simulink model "sim_all"  (R2020a)
settings: Solver=VariableStepAuto  StartTime=0.0  StopTime=2000  RelTol=1e-3
values from neighbouring files (symbols this model uses):
  a1 = rho * D^4 * alpha1    (= 0.000388302366464)    [data_current.m]
  a2 = -rho * D^3 * alpha2 * (1 - omega)    (= 0.0037030698432)    [data_current.m]
  alpha1 = 0.0113    [data_current.m]
  alpha2 = -0.0091    [data_current.m]
  cornerA = [43.781381 ... (first row only)    [missionC.m]
  cornerB = [43.780975 ... (first row only)    [missionC.m]
  cornerC = [43.780189 ... (first row only)    [missionC.m]
  cornerD = [43.780602 ... (first row only)    [missionC.m]
  ctrl_clockwise = false    [controller.m]
  ctrl_int_bound_or = 0.1    [controller.m]
  ctrl_int_bound_pos = 1    [controller.m]
  ctrl_k_or = 1    [controller.m]
  ctrl_k_pos = 1/3    (= 0.333333333333)    [controller.m]
  ctrl_Ki_vel = 100    [controller.m]
  ctrl_Kp_v_pos = 200    [controller.m]
  ctrl_Kp_vel = 200    [controller.m]
  ctrl_TAM = [  1     1           0           0               0       0;               0     0           1           1               0       0;               0     0           0           0               1       1;               0     0  -(ctrl_r+ctrl_dc)  ctrl_r+ctrl_dc    0       0;               0     0           0           0            -ctrl_r    ctrl_r;           -ctrl_r ctrl_r        0           0       ...(+19 chars)    [controller.m]
  ctrl_Ts = 0.1    [controller.m]
  ctrl_va_uncontrolled = 0.15    [controller.m]
  ctrl_vel_uncontrolled = 0.5    [controller.m]
  D = 0.076    [data_current.m]
  dead_zone_limit = 31.5    [data_current.m]
  depth = 5    [missionC.m]
  distanceFromWall = 8    [missionC.m]
  initInspectedSide = 2    [missionC.m]
  initPoint = [ 43.780796 ... (first row only)    [missionC.m]
  mod_A = pi*mod_R*mod_R    [model.m]
  mod_Cd_F = 0.45    [model.m]
  mod_Cd_M = 0.4    [model.m]
  mod_eta_init = [mod_xNorth; mod_yEast; -mod_zDown; 0; 0; 0]    [model.m]
  mod_g = 9.81    [model.m]
  mod_h0 = 0    [model.m]
  mod_Ixx = mod_Io(1,1)    [model.m]
  mod_Iyy = mod_Io(2,2)    [model.m]
  mod_Izz = mod_Io(3,3)    [model.m]
  mod_Kp_dot = 0    [model.m]
  mod_lat0 = 43.780189    [model.m]
  mod_lon0 = 11.282698    [model.m]
  mod_m = 100    [model.m]
  mod_Mq_dot = mod_Kp_dot    (= 0)    [model.m]
  mod_ni_init = [0; 0; 0; 0; 0; 0]    [model.m]
  mod_Nr_dot = mod_Kp_dot    (= 0)    [model.m]
  mod_p1 = [0; mod_R; 0]    [model.m]
  mod_p2 = [0; -mod_R; 0]    [model.m]
  mod_p3 = [0; 0; (mod_R + mod_z_cm)]    [model.m]
  mod_p4 = [0; 0; -(mod_R + mod_z_cm)]    [model.m]
  mod_p5 = [mod_R; 0; 0]    [model.m]
  mod_p6 = [-mod_R; 0; 0]    [model.m]
  mod_R = ((3*mod_Vol)/(4*pi))^(1/3)    [model.m]
  mod_Rm = (4*mod_R)/(3*pi)    [model.m]
  mod_t1 = [1; 0; 0]    [model.m]
  mod_t2 = [1; 0; 0]    [model.m]
  mod_t3 = [0; 1; 0]    [model.m]
  mod_t4 = [0; 1; 0]    [model.m]
  mod_t5 = [0; 0; 1]    [model.m]
  mod_t6 = [0; 0; 1]    [model.m]
  mod_W = mod_m*mod_g    (= 981)    [model.m]
  mod_Xu_dot = (2/3)*mod_rho_AUV*pi*(mod_R^3)    [model.m]
  mod_Yv_dot = mod_Xu_dot    [model.m]
  mod_z_cm = mod_r_cm(3)    [model.m]
  mod_Zw_dot = mod_Xu_dot    [model.m]
  n_max = 340    [data_current.m]
  nav_DT = 0.1    [navigation.m]
  nav_filter = -1    [data_analysis_simulation_total.m]    (also in navigation.m)
  nav_giro = 2    [navigation.m]
  nav_h0 = 0    [navigation.m]
  nav_lat0 = cornerC(1)    [navigation.m]
  nav_lon0 = cornerC(2)    [navigation.m]
  nav_plane_AB = coefficient_plane(nav_A,nav_B)    [navigation.m]
  nav_plane_BC = coefficient_plane(nav_B,nav_C)    [navigation.m]
  nav_plane_CD = coefficient_plane(nav_C,nav_D)    [navigation.m]
  nav_plane_DA = coefficient_plane(nav_D,nav_A)    [navigation.m]
  nav_resampling = 10000    [navigation.m]
  omega = 0.1    [data_current.m]
  relativeDirection = 30    [missionC.m]
  res_enable_n_eff = 1    [navigation.m]
  rho = 1030    [data_current.m]
  sens_distCM = 0.267    [sensors.m]
  sens_Sample_time_AHRS = 0.1    [sensors.m]
  sens_Sample_time_depth = 0.1    [sensors.m]
  sens_Sample_time_dvl = 0.2    [sensors.m]
  sens_Sample_time_GPS = 1    [sensors.m]
  sens_Sample_time_GYRO = 0.1    [sensors.m]
  sens_Sample_time_sonar = 0.5    [sensors.m]
  sens_threshold = 0.485    [sensors.m]
  sens_Variance_AHRS_pitch = (0.0087)^2    (= 7.569e-05)    [sensors.m]
  sens_Variance_AHRS_roll = (0.0087)^2    (= 7.569e-05)    [sensors.m]
  sens_Variance_AHRS_yaw = (0.0017)^2    (= 2.89e-06)    [sensors.m]
  sens_Variance_depth1 = (0.2)^2    (= 0.04)    [sensors.m]
  sens_Variance_depth2 = (0.4)^2    (= 0.16)    [sensors.m]
  sens_Variance_DVL = (speed*0.03)^2    [sensors.m]
  sens_Variance_GPS = 3    [sensors.m]
  sens_Variance_GYRO = 2.5133e-06    [sensors.m]
  sens_Variance_sonar = 0.05    [sensors.m]
  soglia_or = [0.1, 0.1, 0.1]    [mission.m]
  soglia_orp = 0.1    [mission.m]
  soglia_parete = 0.5    [mission.m]
  soglia_parete_frenata = 0.5    [mission.m]
  soglia_pos = [0.00001, 0.00001, 0.5]    [mission.m]
  soglia_SOS_collisione = 2    [mission.m]
  soglia_SOS_or = [0.25, 0.25, 0.25]    [mission.m]
  soglia_SOS_orp = 0.25    [mission.m]
  soglia_SOS_parete = 1    [mission.m]
  soglia_SOS_pos = [0.00005, 0.00005, 1]    [mission.m]
  soglia_SOS_pos_ris = 2    [mission.m]
  soglia_SOS_vel = 0.2    [mission.m]
  SOS = 0    [mission.m]
  speed = 0.4    [missionC.m]
  stato = 100    [mission.m]
  timer = 40*2    (= 80)    [mission.m]
  Ts_supervisor = 0.1    [mission.m]
undefined symbols (not defined in the file or in its folder): DiscIntNeverNeededParam, nav_A, nav_B, nav_C, nav_D
libraries: simulink x8, cstblocks x6, simulink_extras x1
(part 6 of 8)

== matlab function sim_all/Mission_supervisor_v3/Mission_Supervisor/Manovra/MATLAB Function ==
  data: delta_current_man output; delta_stato_man output; contatore output; contatore input; Pos_d output size=3; Dpp_d output; Dps_d output; Orp_d output; Pos_s input; Dpp_s input; Orp_s input; distanceFromWall parameter; relativeDirection parameter; depth parameter; error_flag input; soglia_orp parameter; soglia_SOS_parete parameter; soglia_SOS_pos parameter; SOS parameter; Dps_s input; alfa input; giro input; parete_attuale input
function [delta_current_man, delta_stato_man, contatore, Pos_d, Dpp_d, Dps_d, Orp_d] = Manovra(contatore, Pos_s, Dpp_s, Orp_s, distanceFromWall, relativeDirection, depth, error_flag, soglia_orp, soglia_SOS_parete, soglia_SOS_pos, SOS, Dps_s, alfa, giro, parete_attuale)

    disp("Manovra");
    
    %% Unità di misura 
     
    % Pos_d, Pos_s, soglia_SOS_pos                                                [deg,deg,m]
    % Orp_d, Orp_s, soglia_orp, alfa                                              [rad]
    % relativeDirection                                                           [deg]
    % Dpp_d, Dps_d, Dpp_s, Dps_s, distanceFromWall, depth, soglia_SOS_parete      [m]


    %% Inizializzazione variabili
    
    delta_stato_man = -2 * contatore;
    
    pronti = false;
    
    relativeDirection_rad = deg2rad(relativeDirection);
    
    % Si utilizza la variabile booleana giro, inizializzata nella matlab function "aggiornamento della parete"
    % per determinare il senso di pattugliamento
    if giro == 0 % orario
        inspectionDirection = "clockwise";
    else % antiorario
        inspectionDirection = "counterclockwise";
    end

    %% Preparazione dei riferimenti da fornire si blocchi successivi
          
    Pos_d = [nan; nan; depth];
                                                                            %*****TEST******%
                                                                            %Pos_d = [nan; nan; 0];
    % Distanza dalla parete da mantenere
    Dpp_d = distanceFromWall;
    Dps_d = distanceFromWall;
    
    % Orientazione relativa alla parete
    Orp_d = relativeDirection_rad;
    
    % In questo stato il riferimento di orientazione passato al controllo
    % si riferisce alla parete successiva. Questo rende necessario
    % l'introduzione della variabile "Orp_rif" utilizzata nelle condizioni
    % di switch poiché il valore di stima si riferisce ancora alla parete attuale.
    % I valori alfa corrispondono agli angoli interni ai corner del bacino.
    if (strcmp(inspectionDirection,'clockwise') == 1) % AB-BC-CD-DA
        
        if parete_attuale == 1 % pattugliamento AB, manovra in B
            Orp_rif = relativeDirection_rad + alfa(2); 
        elseif parete_attuale == 2 % pattugliamento BC, manovra in C
            Orp_rif = relativeDirection_rad + alfa(3);
        elseif parete_attuale == 3 % pattugliamento CD, manovra in D
            Orp_rif = relativeDirection_rad + alfa(4);
        else  % pattugliamento DA, manovra in A
            Orp_rif = relativeDirection_rad + alfa(1);
        end
        
    else % AB-DA-CD-BC
        
        if parete_attuale == 1 % pattugliamento AB, manovra in A
            Orp_rif = relativeDirection_rad - alfa(1);
        elseif parete_attuale == 2 % pattugliamento BC, manovra in B
            Orp_rif = relativeDirection_rad - alfa(2);
        elseif parete_attuale == 3 % pattugliamento CD, manovra in C
            Orp_rif = relativeDirection_rad - alfa(3);
        else % pattugliamento DA, manovra in D
            Orp_rif = relativeDirection_rad - alfa(4);
        end
    end
      
    % Transizione di stato effettiva
    delta_current_man = 203 - 202 + contatore;           
    
       
    %% Verifiche
    
    % Verifica di aver mantenuto la corretta profondità e distanza
    % dalle pareti considerate
    if (abs(Pos_s(3) - Pos_d(3)) > soglia_SOS_pos(3) || ...
       abs(Dpp_s - Dpp_d) > soglia_SOS_parete || ...
       abs(Dps_s - Dps_d) > soglia_SOS_parete)
    
        SOS = 1;
        disp("EMERGENZA:");
        
        if (abs(Pos_s(3) - Pos_d(3)) > soglia_SOS_pos(3))
            disp("Rilevato errore sulla profondita");
        end
        if (abs(Dpp_s - Dpp_d) > soglia_SOS_parete)
            disp("Rilevato errore sulla distanza da parete");
        end
        if (abs(Dps_s - Dps_d) > soglia_SOS_parete)
            disp("Rilevato errore sulla distanza da parete successiva");
        end
    end
    
                                                                            %*****TEST******%
                                                                            % if(contatore > 1)
                                                                            %     error_flag = 1;
                                                                            % end

     if error_flag == 1
        disp("EMERGENZA: errore segnalato dagli altri sottosistemi");
        SOS = 1;
     end
     
     
                                                                            %*****TEST******%
                                                                            %Serve per testare di rimanere 
                                                                            %in attesa in questo stato 
                                                                            %test = 0;
                                                                            %if(contatore > 2)%test
                                                                            %    test = 100;
                                                                            %else
                                                                            %    test = 0;
                                                                            %end
                                                                            
    % Si verifica di aver raggiunto l'orientazione desiderata 
    if (SOS == 0 && ...
        abs(Orp_s - Orp_rif) < soglia_orp)    
    
        pronti = true;
        
    end
    
    % La parete viene aggiornata soltanto
    % al termine della fase di manovra incrementando il contatore
    if pronti == true
         contatore = contatore + 1;
    end
    
     
    %% Decisione dello stato successivo
    
    if pronti == true
        if contatore < 4    % Non è ancora il pattugliamento dell'ultima parete 
            
            delta_stato_man = 201 - 203 - 2 * contatore +2;   % Si continua il pattugliamento delle pareti successive  
            
        else    % Completato il pattugliamento dell'ultima parete intera, si esce dal ciclo per
                % effettuare il pattugliamento parziale della parete
                % iniziale che era stata pattugliata solo per metà
                
            delta_stato_man = 204-203 - 2 * contatore +2;         
        end
    end
    
    if SOS == 1
            
            delta_stato_man = 301-203 + - 2 * contatore; %Transizione nello stato di emergenza
    end
        % Si rimane nello stato corrente

end

== matlab function sim_all/Mission_supervisor_v3/Mission_Supervisor/Completamento/MATLAB Function ==
  data: delta_current_comp output; parete input; delta_stato_comp output; Pos_d output size=3; Vel_d output; Dpp_d output; Orp_d output; Pos_s input; Vel_s input; Dpp_s input; Dps_s input; Orp_s input; depth parameter; speed parameter; distanceFromWall parameter; relativeDirection parameter; dps_fin input; error_flag input; soglia_SOS_vel parameter; soglia_parete_frenata parameter; soglia_SOS_orp parameter; soglia_SOS_pos parameter; soglia_SOS_parete parameter; SOS parameter; giro input
function [delta_current_comp, delta_stato_comp, Pos_d, Vel_d, Dpp_d, Orp_d] = Completamento(parete, Pos_s, Vel_s, Dpp_s, Dps_s, Orp_s, depth, speed, distanceFromWall, relativeDirection, dps_fin, error_flag, soglia_SOS_vel, soglia_parete_frenata, soglia_SOS_orp, soglia_SOS_pos, soglia_SOS_parete, SOS, giro)

    disp("Completamento del pattugliamento parziale della parete " + parete);
    
    %% Unità di misura 
    
    % Pos_d, Pos_s, soglia_SOS_pos                                                                              [deg, deg, m]
    % Orp_d, Orp_s, soglia_SOS_orp                                                                              [rad]
    % relativeDirection                                                                                         [deg]
    % Dpp_d, Dps_d, Dpp_s, Dps_s, dps_fin, distanceFromWall, depth, soglia_SOS_parete, soglia_parete_frenata    [m]
    % Vel_d, Vel_s, speed, soglia_SOS_vel                                                                       [m/s]

    %% Inizializzazione variabili
    
    % Utilizzata per permanere in questo stato e inizializzata a zero
    % perché fuori dal ciclo
    delta_stato_comp = 0; 
    
    pronti = false;
    
    
    %% Preparazione dei riferimenti da fornire ai blocchi successivi
    
    % Profondità da mantenere
    Pos_d = [nan; nan; depth];
                                                                            %*****TEST******%
                                                                            %Pos_d = [nan; nan; 0];
    
    % Velocità da raggiungere
    Vel_d = speed;              
                                                                            %*****TEST******%
                                                                            %Vel_d_vett = [0; 0; 0];

    % Distanza dalla parete da mantenere
    Dpp_d = distanceFromWall;
    
    % Orientazione da mantenere
    Orp_d = deg2rad(relativeDirection);
        
    % Transizione di stato effettiva
    delta_current_comp = 204 - 203;  
  
    %% Verifiche
    
    % Verifica sulla corretta profondità, orientazione, distanza dalla parete pattugliata 
    % e velocità
    if (abs(Pos_s(3) - Pos_d(3)) > soglia_SOS_pos(3) || ...
        abs(Orp_s - Orp_d) > soglia_SOS_orp || ...
        abs(Dpp_s - Dpp_d) > soglia_SOS_parete || ...
        norm(Vel_s) - Vel_d > soglia_SOS_vel)
    
        SOS = 1;
        disp("EMERGENZA:");
        
        if (abs(Orp_s - Orp_d) > soglia_SOS_orp)
            disp("Rilevato errore sull'orientazione relativa");
        end
        
        if (abs(Dpp_s - Dpp_d) > soglia_SOS_parete)
            disp("Rilevato errore sulla distanza da parete");
        end
        
        if (abs(Pos_s(3) - Pos_d(3)) > soglia_SOS_pos(3))
            disp("Rilevato errore sulla profondita Z");
        end
        
        if (norm(Vel_s) - Vel_d > soglia_SOS_vel)
            disp("Rilevato errore nella velocita");
        end

    end
    
                                                                            %*****TEST******%
                                                                            % if(contatore > 1)
                                                                            %     error_flag = 1;
                                                                            % end

     if error_flag == 1
        disp("EMERGENZA: errore segnalato dagli altri sottosistemi");
        SOS = 1;
     end
     
                                                                            %*****TEST******%
                                                                            %dps_fin = 4;

    % Si verifica di pattugliare alla velocità desiderata fino al punto di
    % frenata
    if (SOS == 0 && ...
        abs(Dps_s - (dps_fin + 3*speed)) < soglia_parete_frenata) % Analogo a quanto detto in "Pattugliamento"
    
        pronti = true;
        
    end
    
    %% Decisione dello stato successivo
    
    if pronti == true
        
        delta_stato_comp = 205 - 204; % Transizione eseguita correttamente
    end
    if SOS == 1
            
            delta_stato_comp = 301 - 204; % Transizione nello stato di emergenza
    end
  % Si rimane nello stato corrente.

end

== matlab function sim_all/Mission_supervisor_v3/Mission_Supervisor/Frenata in completamento/MATLAB Function ==
  data: delta_current_fren_comp output; delta_stato_fren_comp output; SOS_205 output; Pos_d output size=3; Dpp_d output; Dps_d output; Orp_d output; Pos_s input; Orp_s input; Dpp_s input; Dps_s input; depth parameter; distanceFromWall parameter; relativeDirection parameter; dps_fin input; error_flag input; soglia_SOS_pos parameter; soglia_SOS_parete parameter; soglia_SOS_orp parameter; soglia_parete parameter; SOS parameter
function [delta_current_fren_comp, delta_stato_fren_comp, SOS_205, Pos_d, Dpp_d, Dps_d, Orp_d] = Frenata_completamento(Pos_s, Orp_s, Dpp_s, Dps_s, depth, distanceFromWall, relativeDirection, dps_fin, error_flag, soglia_SOS_pos, soglia_SOS_parete, soglia_SOS_orp, soglia_parete, SOS)

    disp("Frenata (durante il completamento del pattugliamento parziale)");
    
    %% Unità di misura 
    
    % Pos_d, Pos_s, soglia_SOS_pos                                                                      [deg, deg, m]
    % Orp_d, Orp_s, soglia_SOS_orp                                                                      [rad]
    % relativeDirection                                                                                 [deg]
    % Dpp_d, Dps_d, Dpp_s, Dps_s, dps_fin, distanceFromWall, depth, soglia_SOS_parete, soglia_parete    [m]
    
    %% Inizializzazione variabili
    
    delta_stato_fren_comp = 0;
    
    pronti = false;
    

    %% Preparazione dei riferimenti da fornire si blocchi successivi
    
    % Profondità da mantenere
    Pos_d = [nan; nan; depth];
                                                                            %*****TEST******%
                                                                            %Pos_d = [nan;nan;0];
    % Distanza dalla parete da mantenere
    Dpp_d = distanceFromWall;
    Dps_d = dps_fin;
    
    % Orientazione da mantenere
    Orp_d = deg2rad(relativeDirection);
    
    % Transizione di stato effettiva
    delta_current_fren_comp = 205 - 204;  
    
       
    %% Verifiche

    % Si verifica la corretta orientazione, profondità e distanza dalla parete di pattugliamento 
    if (abs(Pos_s(3) - Pos_d(3)) > soglia_SOS_pos(3) || ...
        abs(Orp_s - Orp_d) > soglia_SOS_orp || ...
        abs(Dpp_s - Dpp_d) > soglia_SOS_parete)
    
        SOS = 1;
        pronti = true;
        disp("EMERGENZA:");
        
        if (abs(Pos_s(3) - Pos_d(3)) > soglia_SOS_pos(3))
            disp("Rilevato errore sulla profondita Z");
        end
        
        if (abs(Orp_s - Orp_d) > soglia_SOS_orp)
            disp("Rilevato errore sull'orientazione relativa");
        end
        
        if (abs(Dpp_s - Dpp_d) > soglia_SOS_parete)
            disp("Rilevato errore sulla distanza da parete");
        end
    end
    
    if error_flag == 1
        disp("EMERGENZA: errore segnalato dagli altri sottosistemi");
        SOS = 1;
    end
 
    SOS_205 = SOS;                                                                     %*****TEST******%
                                                                            %dps_fin = 8;

    % Si verifica di aver raggiunto la posizione desiderata di fine pattugliamento
    if (SOS==0 && ...
        abs(Dps_s - dps_fin) < soglia_parete) 
        pronti = true;
        
    end
    
    %% Decisione dello stato successivo
    
    if (pronti == true || SOS == 1)
        
        delta_stato_fren_comp = 301 - 205; % Transizione di stato
    end
    % Si rimane nello stato corrente
    

end

== matlab function sim_all/Mission_supervisor_v3/Mission_Supervisor/Orientazione in superficie/MATLAB Function ==
  data: delta_current_or_sup output; delta_stato_or_sup output; Or_in input; error_flag input; punto_iniz_patt input; SOS parameter; Pos_d output size=3; Or_d output size=3; soglia_SOS_pos parameter; soglia_or parameter; Pos_s input; Or_s input; soglia_SOS_or parameter
function [delta_current_or_sup, delta_stato_or_sup, Pos_d, Or_d] = Orientazioneinsuperficie(Or_in, error_flag, punto_iniz_patt, SOS, soglia_SOS_pos, soglia_or, Pos_s, Or_s, soglia_SOS_or)

    disp("Orientazione in superficie");
    
    %% Unità di misura 
    
    % Pos_d, Pos_s, soglia_SOS_pos, punto_iniz_patt                             [deg,deg,m]
    % Or_d, Or_in, Or_s, soglia_SOS_or, soglia_or                               [deg,deg,deg]

    %% Inizializzazione variabili
    
    delta_stato_or_sup = 0;
    
    pronti = false; 

    %% Preparazione dei riferimenti da fornire ai blocchi successivi
  
    % Posizione da mantenere
    Pos_d = punto_iniz_patt; 
                                                                            %*****TEST******%
                                                                            %Pos_d = [43; 11; 0];  
    % Orientazione desiderata e necessaria per raggiungere
    % il punto di rientro
    Or_d = Or_in;
                                                                            %*****TEST******%
                                                                            %Or_d = [1; 1; 1];
  
    % Transizione di stato effettiva
    delta_current_or_sup = 302 - 301;
   
    
    %% Verifiche 
    
    % Verifica della posizione e dell'orientazione
   if (abs(Pos_s(1) - Pos_d(1)) > soglia_SOS_pos(1) || ...
       abs(Pos_s(2) - Pos_d(2)) > soglia_SOS_pos(2) || ...
       abs(Pos_s(3) - Pos_d(3)) > soglia_SOS_pos(3) || ...
       abs(Or_s(1) - Or_d(1)) > soglia_SOS_or(1) || ...
       abs(Or_s(2) - Or_d(2)) > soglia_SOS_or(2))
    
        SOS = 1;
        disp("EMERGENZA:");
        
        
        if (abs(Pos_s(1) - Pos_d(1)) > soglia_SOS_pos(1))
            disp("Rilevato errore sulla posizione X");
        end
        if (abs(Pos_s(2) - Pos_d(2)) > soglia_SOS_pos(2))
            disp("Rilevato errore sulla posizione Y");
        end
        if (abs(Pos_s(3) - Pos_d(3)) > soglia_SOS_pos(3))
            disp("Rilevato errore sulla profondita Z");
        end
        if (abs(Or_s(1) - Or_d(1)) > soglia_SOS_or(1))
            disp("Rilevato errore sulla rotazione di roll");
        end
        if (abs(Or_s(2) - Or_d(2)) > soglia_SOS_or(2))
            disp("Rilevato errore sulla rotazione di pitch");
        end

    end
    
    if error_flag == 1
        disp("EMERGENZA: errore segnalato dagli altri sottosistemi");
        SOS = 1;
    end
    
    % Si verifica di aver raggiunto l'orientazione desiderata
    if  (SOS == 0 && ...
         abs(Or_s(3) - Or_d(3)) < soglia_or(3))
    
        pronti = true;
        
    end
    
%% Decisione dello stato successivo
    
    if pronti == true
       
        delta_stato_or_sup = 303 - 302; % Transizione eseguita correttamente
    end
    
    if SOS == 1
            
            delta_stato_or_sup = 304 - 302; % Transizione nello stato di emergenza
    end

    % Si rimane nello stato corrente
end

== matlab function sim_all/Mission_supervisor_v3/Mission_Supervisor/Pattugliamento/MATLAB Function ==
  data: parete input; contatore input; delta_current_patt output; Pos_s input; Dpp_s input; Dps_s input; delta_stato_patt output; Pos_d output size=3; Vel_d output; Dpp_d output; Orp_d output; Orp_s input; Vel_s input; depth parameter; speed parameter; distanceFromWall parameter; relativeDirection parameter; soglia_parete_frenata parameter; soglia_SOS_orp parameter; soglia_SOS_parete parameter; soglia_SOS_pos parameter; error_flag input; SOS parameter; soglia_SOS_vel parameter; giro input
function [delta_current_patt, delta_stato_patt, Pos_d, Vel_d, Dpp_d, Orp_d] = Pattugliamento(parete, contatore, Pos_s, Dpp_s, Dps_s, Orp_s, Vel_s, depth, speed, distanceFromWall, relativeDirection, soglia_parete_frenata, soglia_SOS_orp, soglia_SOS_parete, soglia_SOS_pos, error_flag, SOS, soglia_SOS_vel, giro)
    
    % In base al valore del contatore un display mostra il tipo di pattugliamento (parziale o completo)
    if contatore == 0
        disp("Pattugliamento parziale parete " + parete);
    else
        disp("Pattugliamento parete " + parete);
    end 
    
    %% Unità di misura 
    
    % Pos_d, Pos_s, soglia_SOS_pos                                                        [deg, deg, m]
    % Orp_d, Orp_s, soglia_SOS_orp                                                        [rad]
    % relativeDirection                                                                   [deg]
    % Dpp_d,Dpp_s, depth, distanceFromWall, soglia_parete_frenata, soglia_SOS_parete      [m]
    % Vel_d, Vel_s, speed, soglia_SOS_vel                                                 [m/s]

    
    %% Inizializzazione variabili
    
    % Si attribuisce alla variabile delta_stato_patt il valore contatore per  
    % tenere traccia delle transizioni effettuate durante il ciclo di
    % pattugliamento. Questo deve essere fatto perché i valori delta_stato
    % rimangono attivi una volta inizializzati nel ciclo.
    delta_stato_patt = contatore;
    
    pronti = false;
    
    %% Preparazione dei riferimenti da fornire ai blocchi successivi
    
    % Profondità da mantenere
    Pos_d = [nan; nan; depth];
                                                                            %*****TEST******%
                                                                            %Pos_d = [nan;nan;0];
    
    % Velocità da raggiungere
    Vel_d = speed;             

    % Distanza dalla parete da mantenere
    Dpp_d = distanceFromWall;
    
    % Orientazione da mantenere
    Orp_d = deg2rad(relativeDirection);
    
    
    % Transizione di stato effettiva a seconda che si arrivi da
    % "Orientazione in profondità" o da "Manovra"
    delta_current_patt = 201-104;   
   
    if contatore>0
        delta_current_patt = 201 - 104 - (2*contatore); 
    end
       
    %% Verifiche
    
    %Verifica sull'orientazione, sulla velocità, sulla profondità e sulla
    %distanza dalla parete pattugliata
    if (abs(Pos_s(3) - Pos_d(3)) > soglia_SOS_pos(3) || ...
        abs(Orp_s - Orp_d) > soglia_SOS_orp || ...
        norm(Vel_s) - Vel_d > soglia_SOS_vel || ...
        abs(Dpp_s - Dpp_d) > soglia_SOS_parete)
 
        SOS = 1;
        disp("EMERGENZA:");
        
        if (abs(Orp_s-Orp_d) > soglia_SOS_orp)
            disp("Rilevato errore sull'orientazione relativa");
        end
        if (abs(Dpp_s - Dpp_d) > soglia_SOS_parete)
            disp("Rilevato errore sulla distanza da parete");
        end
        if (abs(Pos_s(3) - Pos_d(3)) > soglia_SOS_pos(3))
            disp("Rilevato errore sulla profondita");
        end
        if (norm(Vel_s) - Vel_d > soglia_SOS_vel)
            disp("Rilevato errore sulla velocita");
        end

    end
%                                                                             %*****TEST******%
%                                                                             if(contatore>1)
%                                                                                 error_flag=1;
%                                                                             end

     if error_flag == 1
        disp("EMERGENZA: errore segnalato dagli altri moduli");
        SOS = 1;
     end
                                                                            %*****TEST******%
                                                                            %Serve per testare di rimanere 
                                                                            %in attesa in questo stato 
                                                                            %test=0;
%                                                                             if(contatore>1)%test
%                                                                                test=100;
%                                                                             else
%                                                                                test=0;
%                                                                             end
    
    % Si verifica di pattugliare fino al punto di frenata calcolata
    % considerando un tempo di frenata di tre secondi
    if (SOS == 0 && ...
        abs(Dps_s - (distanceFromWall + 3*speed)) < soglia_parete_frenata) 

        
        pronti = true;
        
    end
    
    %% Decisione dello stato successivo
    
    if pronti == true

        delta_stato_patt = 202 - 201 + contatore; %Transizione eseguita correttamente
    end
    if SOS == 1
            
            delta_stato_patt = 301 - 201 + contatore; %Transizione nello stato di emergenza
    end
% Si rimane nello stato corrente

end

== matlab function sim_all/Mission_supervisor_v3/Mission_Supervisor/Fine missione/MATLAB Function ==
  data: delta_current_end output; stato input
function delta_current_end  = Fine_missione(stato)

    disp("Fine missione");
    
    
    
    %% Transizione di stato effettiva 
    delta_current_end = 304 - stato;  
    
    % La missione è conclusa e la simulazione termina.

end

== matlab function sim_all/Mission_supervisor_v3/Mission_Supervisor/Posizionamento/MATLAB Function ==
  data: delta_current_posiz output; delta_stato_posiz output; Pos_d output size=3; Or_d output size=3; Pos_s input; Or_s input; punto_iniziale input; Or_in input; error_flag input; soglia_pos parameter; soglia_SOS_or parameter; SOS parameter; soglia_SOS_pos parameter
function [delta_current_posiz, delta_stato_posiz, Pos_d, Or_d] = Posizionamento(Pos_s, Or_s, punto_iniziale, Or_in, error_flag, soglia_pos, soglia_SOS_or, SOS, soglia_SOS_pos)

    disp("Posizionamento");
    
    %% Unità di misura 
    
    % Pos_d, Pos_s, punto_iniziale, soglia_pos, soglia_SOS_pos             [deg, deg, m]
    % Or_d, Or_s, Or_in, soglia_SOS_or                                     [rad, rad, rad]

    %% Inizializzazione variabili
    
    % Mantenimento dello stato_interno al valore
    % desiderato durante la permanenza del sistema nello stato corrente.
    delta_stato_posiz = 0;
    
    pronti = false;
   
    %% Preparazione dei riferimenti da fornire ai blocchi successivi
    
    % Posizione da raggiungere
    Pos_d = punto_iniziale;                                                %*****TEST******%
                                                                            %Pos_d = [43; 11; 0];
     
   
    % Orientazione da mantenere
    Or_d = Or_in;
    
    % Transizione di stato effettiva
    delta_current_posiz = 102 - 101;  
       
    
    %% Verifiche
    
     % Verifica della corretta orientazione e profondità
     
    if (abs(Or_s(1) - Or_d(1)) > soglia_SOS_or(1) || ...
        abs(Or_s(2) - Or_d(2)) > soglia_SOS_or(2) || ...
        abs(Or_s(3) - Or_d(3)) > soglia_SOS_or(3) || ...
        abs(Pos_s(3) - Pos_d(3)) > soglia_SOS_pos(3))
    
        SOS = 1;
        disp("EMERGENZA:");       
        
        if (abs(Or_s(1) - Or_d(1)) > soglia_SOS_or(1))
            disp("Rilevato errore sulla rotazione di roll");
        end
        
        if (abs(Or_s(2) - Or_d(2)) > soglia_SOS_or(2))
            disp("Rilevato errore sulla rotazione di pitch");
        end
        
        if (abs(Or_s(3) - Or_d(3)) > soglia_SOS_or(3))
            disp("Rilevato errore sulla rotazione di yaw");
        end
       
        if (abs(Pos_s(3) - Pos_d(3)) > soglia_SOS_pos(3))
            disp("Rilevato errore sulla posizione lungo z");
        end
        
    end
    
    if error_flag == 1
        disp("EMERGENZA: errore segnalato dagli altri sottosistemi");
        SOS = 1;
    end
    
    % Si verifica di aver raggiunto la posizione desiderata
    if (SOS == 0 && ...
        abs(Pos_s(1) - Pos_d(1)) < soglia_pos(1) && ...
        abs(Pos_s(2) - Pos_d(2)) < soglia_pos(2))
    
        pronti = true;
        
    end

    %% Decisione dello stato successivo
     
    if pronti == true
        
        delta_stato_posiz = 103 - 102; % Transizione eseguita correttamente
    end
    if SOS == 1
            
            delta_stato_posiz = 304 - 102; % Transizione nello stato di emergenza
    end
    % Si rimane nello stato corrente

end

== matlab function sim_all/Mission_supervisor_v3/Mission_Supervisor/Rientro/MATLAB Function ==
  data: delta_current_rient output; delta_stato_rient output; Pos_d output size=3; Pos_s input; initPoint parameter; Or_in input; Or_d output size=3; soglia_pos parameter; SOS parameter; error_flag input; Dps_s input; Dpp_s input; soglia_SOS_collisione parameter; soglia_SOS_or parameter; soglia_SOS_pos parameter; Or_s input
function [delta_current_rient, delta_stato_rient, Pos_d, Or_d] = Rientro(Pos_s, initPoint, Or_in, soglia_pos, SOS, error_flag, Dps_s, Dpp_s, soglia_SOS_collisione, soglia_SOS_or, soglia_SOS_pos, Or_s)

    disp("Rientro");
    
    %% Unità di misura 
    
    % Pos_d, Pos_s, soglia_pos, initPoint, soglia_SOS_pos                    [deg,deg,m]
    % Or_d, Or_in, Or_s, soglia_SOS_or                                       [deg,deg,deg]
    % Dps_s, Dpp_s, soglia_SOS_collisione_s                                  [m]

    %% Inizializzazione variabili
    
    delta_stato_rient = 0;
    
    pronti = false;
    
    %% Preparazione dei riferimenti da fornire ai blocchi successivi
      
    % Posizione da raggiungere
    Pos_d = initPoint;
    
    % Orientazione da mantenere
    Or_d = Or_in;
    
    % Transizione di stato effettiva
    delta_current_rient = 303 - 302; 
       
    %% Verifiche
    
    % Verifica sulla profondità, sull'orientazione e sull'assenza di collisioni
    if (Dpp_s  < soglia_SOS_collisione || ... 
        Dps_s < soglia_SOS_collisione || ...
        abs(Or_s(1) - Or_d(1)) > soglia_SOS_or(1) || ...
        abs(Or_s(2) - Or_d(2)) > soglia_SOS_or(2) || ...
        abs(Or_s(3) - Or_d(3)) > soglia_SOS_or(3) || ...
        abs(Pos_s(3) - Pos_d(3)) > soglia_SOS_pos(3))
            
    
        SOS = 1;
        disp("EMERGENZA:");  
 

        if (Dpp_s < soglia_SOS_collisione || ... 
            Dps_s < soglia_SOS_collisione)
            disp("Pericolo collisione");
        end
        
        if (abs(Or_s(1) - Or_d(1)) > soglia_SOS_or(1))
            disp("Rilevato errore sulla rotazione di roll");
        end
        
        if (abs(Or_s(2) - Or_d(2)) > soglia_SOS_or(2))
            disp("Rilevato errore sulla rotazione di pitch");
        end
        
        if (abs(Or_s(3) - Or_d(3)) > soglia_SOS_or(3))
            disp("Rilevato errore sulla rotazione di yaw");
        end
     
        if (abs(Pos_s(3) - Pos_d(3)) > soglia_SOS_pos(3))
            disp("Rilevato errore sulla posizione lungo z");
        end
    
    end
    
    if error_flag == 1
        
        disp("EMERGENZA: errore segnalato dagli altri sottosistemi");
        SOS = 1;
        
    end
   
    % Si verifica di aver raggiunto la posizione desiderata
    if (SOS == 0 && ...
        abs(Pos_s(1) - Pos_d(1)) < soglia_pos(1) && ...
        abs(Pos_s(2) - Pos_d(2)) < soglia_pos(2))
    
        pronti = true;
        
    end
    

    
   %% Decisione dello stato successivo
    
   % Si effettua la transizione nello stato successivo indipendentemente
   % dal verificarsi di una emergenza
    if (pronti == true || SOS == 1)

        delta_stato_rient = 304 - 303;
    end
    % Si rimane nello stato corrente

end

== matlab function sim_all/PF/Calcolo distaza pareti/Calcolo distanza dalle pareti ==
  data: pos_es input; dpp output; dps output; parete_attuale input; nav_plane_AB parameter; nav_plane_BC parameter; nav_plane_CD parameter; nav_plane_DA parameter; nav_giro parameter
% Applicando la formula della distanza di un punto da un piano ottengo la
% distanza della posizione dell'AUV dalla parete d'interesse. 

function [dpp,dps] = dpp_dps_calculator(pos_es, parete_attuale, nav_plane_AB, nav_plane_BC, nav_plane_CD, nav_plane_DA, nav_giro)
    
%selezione della parete di pattugliamento e successiva
    switch parete_attuale
        
        case 1
           coef = nav_plane_AB;            %parete attuale AB
           if nav_giro == 1
               coef_succ = nav_plane_BC;   %parete succ BC
           else
               coef_succ = nav_plane_DA;   %parete succ DA
           end
           
        case 2
           coef = nav_plane_BC;            %parete attuale BC
           if nav_giro == 1
               coef_succ = nav_plane_CD;   %parete succ CD
           else
               coef_succ = nav_plane_AB;   %parete succ AB
           end
           
        case 3
           coef = nav_plane_CD;            %parete attuale CD
           if nav_giro == 1
               coef_succ = nav_plane_DA;   %parete succ DA
           else
               coef_succ = nav_plane_BC;   %parete succ BC
           end
        case 4
           coef = nav_plane_DA;            %parete attuale DA
           if nav_giro == 1
               coef_succ = nav_plane_AB;   %parete succ AB
           else
               coef_succ = nav_plane_CD;   %parete succ CD
           end
        otherwise
            coef = [0 0 0 0];
            coef_succ = [0 0 0 0];
    end

    dpp = abs(coef(1)*pos_es(1)+coef(2)*pos_es(2)-coef(3)*pos_es(3)+coef(4))/norm([coef(1) coef(2) coef(3)]);
    dps = abs(coef_succ(1)*pos_es(1)+coef_succ(2)*pos_es(2)-coef_succ(3)*pos_es(3)+coef_succ(4))/norm([coef_succ(1) coef_succ(2) coef_succ(3)]);
   
end

== matlab function sim_all/PF/Calcolo distaza pareti/Calcolo orientazione dalla parete ==
  data: pos_es input; orient_parete output; parete_attuale input; orient input; nav_plane_AB parameter; nav_plane_BC parameter; nav_plane_CD parameter; nav_plane_DA parameter
function orient_parete  = orient_parete_calculator(pos_es, parete_attuale, orient, nav_plane_AB, nav_plane_BC, nav_plane_CD, nav_plane_DA)
    
    %consideriamo angoli di pitch e roll nulli, cioè calcoliamo
    %l'orientazione rispetto alla parete solo considerando rotazioni di yaw
    %(piano xy)

    Yaw   = orient(3);
    R_z = [cos(Yaw)     sin(Yaw)       0     ;
           -sin(Yaw)    cos(Yaw)       0     ;
              0            0           1    ];
    v_pos= R_z'*[1 0 0]';  %versore della retta lungo l'asse x (in body) in NED,
                       %cioè la direzione di riferimento di prua del veicolo     
    
    %selezione della parete di pattugliamento
switch parete_attuale                      
    case 1
        %% Piano di pattugliamento AB
        versore_plane_NED = [nav_plane_AB(1) nav_plane_AB(2) 0]';    %versore normale al piano
        versore_plane_NED = versore_plane_NED/norm(versore_plane_NED);

        %calcolo distanza e intersezione lungo la normale al piano
        t_ = -(pos_es(1)+nav_plane_AB(2)*pos_es(2)+nav_plane_AB(4))/(nav_plane_AB(2)*versore_plane_NED(2)+versore_plane_NED(1));
        inter_perp=zeros(3,1);
        inter_perp(1) = pos_es(1) + versore_plane_NED(1)*t_;
        inter_perp(2) = pos_es(2) + versore_plane_NED(2)*t_;
        inter_perp(3) = pos_es(3) + versore_plane_NED(3)*t_;
        
        %calcolo distanza e intersezione lungo la direzione di prua
        t_ = -(pos_es(1)+nav_plane_AB(2)*pos_es(2)+nav_plane_AB(4))/(nav_plane_AB(2)*v_pos(2)+v_pos(1));
        inter_prua=zeros(3,1);
        inter_prua(1) = pos_es(1) + v_pos(1)*t_;
        inter_prua(2) = pos_es(2) + v_pos(2)*t_;
        inter_prua(3) = pos_es(3) + v_pos(3)*t_;
        
        coef = nav_plane_AB;
        coef(4)=[];
        orient_parete = rad2deg(asin(abs(coef*v_pos)/(norm(coef)*norm(v_pos))));
        %se orient_parete è positiva, allora ci troviamo tra - 90 e + 90 rispetto alla normale della parete 
        if t_ > 0              
            if inter_prua(1) > inter_perp(1) && inter_prua(2) < inter_perp(2)
                orient_parete = orient_parete - 90;
            else
                orient_parete = -(orient_parete - 90);
            end
        else
            if inter_prua(1) > inter_perp(1) && inter_prua(2) < inter_perp(2)
                orient_parete = (orient_parete + 90);
            else
                orient_parete = -(orient_parete + 90);
            end
        end    
    case 2
        %% Piano di pattugliamento BC
      	versore_plane_NED = [nav_plane_BC(1) nav_plane_BC(2) 0]';    %versore normale al piano
        versore_plane_NED = versore_plane_NED/norm(versore_plane_NED);

        %calcolo distanza e intersezione lungo la normale al piano
        t_ = -(pos_es(1)+nav_plane_BC(2)*pos_es(2)+nav_plane_BC(4))/(nav_plane_BC(2)*versore_plane_NED(2)+versore_plane_NED(1));
        inter_perp=zeros(3,1);
        inter_perp(1) = pos_es(1) + versore_plane_NED(1)*t_;
        inter_perp(2) = pos_es(2) + versore_plane_NED(2)*t_;
        inter_perp(3) = pos_es(3) + versore_plane_NED(3)*t_;

        %calcolo distanza e intersezione lungo la direzione di prua
        t_ = -(pos_es(1)+nav_plane_BC(2)*pos_es(2)+nav_plane_BC(4))/(nav_plane_BC(2)*v_pos(2)+v_pos(1));
        inter_prua=zeros(3,1);
        inter_prua(1) = pos_es(1) + v_pos(1)*t_;
        inter_prua(2) = pos_es(2) + v_pos(2)*t_;
        inter_prua(3) = pos_es(3) + v_pos(3)*t_;
        
        coef = nav_plane_BC;
        coef(4)=[];
        v_pos=-v_pos;
        orient_parete = rad2deg(asin(abs(coef*v_pos)/(norm(coef)*norm(v_pos))));
        %se orient_parete è positiva, allora ci troviamo tra - 90 e + 90 rispetto alla normale della parete 
        if t_ > 0              
            if inter_prua(1) > inter_perp(1) && inter_prua(2) > inter_perp(2)
                orient_parete = orient_parete - 90;
            else
                orient_parete = -(orient_parete - 90);
            end
        else
            if inter_prua(1) > inter_perp(1) && inter_prua(2) > inter_perp(2)
                orient_parete = orient_parete + 90;
            else
                orient_parete = -(orient_parete + 90);
            end
        end
        
    case 3
        %% Piano di pattugliamento CD
      	versore_plane_NED = [nav_plane_CD(1) nav_plane_CD(2) 0]';    %versore normale al piano
        versore_plane_NED = versore_plane_NED/norm(versore_plane_NED);

        %calcolo distanza e intersezione lungo la normale al piano
        t_ = -(pos_es(1)+nav_plane_CD(2)*pos_es(2)+nav_plane_CD(4))/(nav_plane_CD(2)*versore_plane_NED(2)+versore_plane_NED(1));
        inter_perp=zeros(3,1);
        inter_perp(1) = pos_es(1) + versore_plane_NED(1)*t_;
        inter_perp(2) = pos_es(2) + versore_plane_NED(2)*t_;
        inter_perp(3) = pos_es(3) + versore_plane_NED(3)*t_;

        %calcolo distanza e intersezione lungo la direzione di prua
        t_ = -(pos_es(1)+nav_plane_CD(2)*pos_es(2)+nav_plane_CD(4))/(nav_plane_CD(2)*v_pos(2)+v_pos(1));
        inter_prua=zeros(3,1);
        inter_prua(1) = pos_es(1) + v_pos(1)*t_;
        inter_prua(2) = pos_es(2) + v_pos(2)*t_;
        inter_prua(3) = pos_es(3) + v_pos(3)*t_;
        
        coef = nav_plane_CD;
        coef(4)=[];
        v_pos=-v_pos;
        orient_parete = rad2deg(asin(abs(coef*v_pos)/(norm(coef)*norm(v_pos))));
        %se orient_parete è positiva, allora ci troviamo tra - 90 e + 90 rispetto alla normale della parete 
        if t_ > 0              
            if inter_prua(1) > inter_perp(1) && inter_prua(2) < inter_perp(2)
                orient_parete = -orient_parete + 90;
            else
                orient_parete = orient_parete - 90;
            end
        else
             if inter_prua(1) > inter_perp(1) && inter_prua(2) < inter_perp(2)
                orient_parete = -orient_parete - 90;
            else
                orient_parete = orient_parete + 90;
            end
        end
        
    case 4
        %% Piano di pattugliamento DA
      	versore_plane_NED = [nav_plane_DA(1) nav_plane_DA(2) 0]';    %versore normale al piano
        versore_plane_NED = versore_plane_NED/norm(versore_plane_NED);

        %calcolo distanza e intersezione lungo la normale al piano
        t_ = -(pos_es(1)+nav_plane_DA(2)*pos_es(2)+nav_plane_DA(4))/(nav_plane_DA(2)*versore_plane_NED(2)+versore_plane_NED(1));
        inter_perp=zeros(3,1);
        inter_perp(1) = pos_es(1) + versore_plane_NED(1)*t_;
        inter_perp(2) = pos_es(2) + versore_plane_NED(2)*t_;
        inter_perp(3) = pos_es(3) + versore_plane_NED(3)*t_;

        %calcolo distanza e intersezione lungo la direzione di prua
        t_ = -(pos_es(1)+nav_plane_DA(2)*pos_es(2)+nav_plane_DA(4))/(nav_plane_DA(2)*v_pos(2)+v_pos(1));
        inter_prua=zeros(3,1);
        inter_prua(1) = pos_es(1) + v_pos(1)*t_;
        inter_prua(2) = pos_es(2) + v_pos(2)*t_;
        inter_prua(3) = pos_es(3) + v_pos(3)*t_;
        
        coef = nav_plane_DA;
        coef(4)=[];
        orient_parete = rad2deg(asin(abs(coef*v_pos)/(norm(coef)*norm(v_pos))));
        %se orient_parete è positiva, allora ci troviamo tra - 90 e + 90 rispetto alla normale della parete 
        if t_ > 0              
            if inter_prua(1) < inter_perp(1) && inter_prua(2) < inter_perp(2)
                orient_parete = orient_parete - 90;
            else
                orient_parete = -orient_parete + 90;
            end
        else
            if inter_prua(1) < inter_perp(1) && inter_prua(2) < inter_perp(2)
                orient_parete = orient_parete + 90;
            else
                orient_parete = -orient_parete - 90;
            end
        end
        
    otherwise
        %%
       coef=[0 0 0 0];
       orient_parete = NaN;
end
    
    
end

== matlab function sim_all/PF/ECEF2NED ==
  data: GPS_ECEF input; GPS_NED output; nav_lat0 parameter; nav_lon0 parameter; nav_h0 parameter
%Componente di ingresso in terna ECEF
%Lat  [gradi]
%Long  [gradi]
%flag data_valid

function GPS_NED = GPS_conv_valid(GPS_ECEF, nav_lat0, nav_lon0, nav_h0)
    
    coder.extrinsic('evalin', 'wgs84Ellipsoid', 'geodetic2ned');

    if GPS_ECEF(3)==1
        GPS_NED = zeros(3,1);
        [GPS_NED(1),GPS_NED(2),GPS_NED(3)]= geodetic2ned(GPS_ECEF(1),GPS_ECEF(2),0,nav_lat0,nav_lon0,nav_h0,wgs84Ellipsoid);
        GPS_NED(3) = GPS_ECEF(3);
    else                            %qui ci risparmiamo la conversione se il dato non è valido
        GPS_NED = GPS_ECEF; 
    end
end

== matlab function sim_all/Controller_mk4_v3/C_or/C_or_X ==
  data: err_int output; ang input; vel output; k input; ctrl_va_uncontrolled parameter; ctrl_int_bound_or parameter
%% Azione proporzionale
function [err_int, vel] = fcn(ang, k, ctrl_va_uncontrolled, ctrl_int_bound_or)
    v = 0;
    err_int = 0;
    va_des = ctrl_va_uncontrolled;  % velocità impostata prima della fase di frenata
    brake_dist = (1/k)*va_des;      % distanza in cui dobbiamo iniziare a frenare
    if ang >= brake_dist            % al di fuori dello spazio di frenata
        v = va_des;
    end
    if ang <= -brake_dist           % al di fuori dello spazio di frenata in negativo
        v = -va_des;
    end
    if  abs(ang) < brake_dist       % proporzionale se entro la distanza di frenata
        v = k*ang;
    end
    vel = v;
    if abs(ang) < ctrl_int_bound_or    % per il regime può essere utile una azione integrale
        err_int = ang;                 % err_int va ad un integratore
    end
end

== matlab function sim_all/Controller_mk4_v3/C_or/C_or_Y ==
  data: err_int output; ang input; vel output; k input; ctrl_va_uncontrolled parameter; ctrl_int_bound_or parameter
%% Azione proporzionale
function [err_int, vel] = fcn(ang, k, ctrl_va_uncontrolled, ctrl_int_bound_or)
    v = 0;
    err_int = 0;
    va_des = ctrl_va_uncontrolled;  % velocità impostata prima della fase di frenata
    brake_dist = (1/k)*va_des;      % distanza in cui dobbiamo iniziare a frenare
    if ang >= brake_dist            % al di fuori dello spazio di frenata
        v = va_des;
    end
    if ang <= -brake_dist           % al di fuori dello spazio di frenata in negativo
        v = -va_des;
    end
    if  abs(ang) < brake_dist       % proporzionale se entro la distanza di frenata
        v = k*ang;
    end
    vel = v;
    if abs(ang) < ctrl_int_bound_or    % per il regime può essere utile una azione integrale
        err_int = ang;                 % err_int va ad un integratore
    end
end
